simulink model "RB_KAIROS_impControl_compensation"  (R2020b)
settings: Solver=ode4  StartTime=0.0  StopTime=t_end  FixedStep=Ts  RelTol=1e-3
values from neighbouring files (symbols this model uses):
  am = 0.3    [RB_KAIROS_ImpControl_OpSpace_quat_2020b_safety_main.m]
  am_r = 0.3    [RB_KAIROS_ImpControl_OpSpace_quat_2020b_safety_main.m]
  Kc = diag(50*ones(6,1))    [RB_KAIROS_ImpControl_OpSpace_quat_2020b_safety_main.m]
  Kp = 2*[400;400;400;400;0;0;0]    [RB_KAIROS_ImpControl_OpSpace_quat_2020b_safety_main.m]
  Kv = [1000;1000;1000;[300;300;300;300;300;300;300]]    [RB_KAIROS_ImpControl_OpSpace_quat_2020b_safety_main.m]
  model_sample_time = 0.001    [RB_KAIROS_ImpControl_OpSpace_quat_2020b_safety_main.m]
  q_dot_0 = zeros(10,1)    [RB_KAIROS_ImpControl_OpSpace_quat_2020b_safety_main.m]
  T_i = K    [RB_KAIROS_ImpControl_OpSpace_quat_2020b_safety_main.m]
  tau_ext = [0 0 0 0 0 0 0 0 0 0 0]    [RB_KAIROS_ImpControl_OpSpace_quat_2020b_safety_main.m]
  v_SMU = 10    [RB_KAIROS_ImpControl_OpSpace_quat_2020b_safety_main.m]
  vm = 0.5    [RB_KAIROS_ImpControl_OpSpace_quat_2020b_safety_main.m]
  vm_r = 0.5    [RB_KAIROS_ImpControl_OpSpace_quat_2020b_safety_main.m]
undefined symbols (not defined in the file or in its folder): DiscIntNeverNeededParam, magnitude, q_0, T_f
libraries: simulink x4, utils x4, transformations_lib x3
(part 11 of 18)

== matlab function RB_KAIROS_impControl_compensation/CONTROLLER /Kinematics and Dynamics/Dynamics - Configuration space/Arm Gravity terms ==
  data: qv input; G output; qa input; g input
function G = get_G(qv,qa,g)
%GET_G
%    G = GET_G(qv,qa,G)

%    This function was generated by the Symbolic Math Toolbox version 8.6.
%    14-Feb-2023 10:02:51

q2 = qa(2);
q3 = qa(3);
q4 = qa(4);
q5 = qa(5);
q6 = qa(6);
q7 = qa(7);
t2 = cos(q2);
t3 = cos(q3);
t4 = cos(q4);
t5 = cos(q5);
t6 = cos(q6);
t7 = cos(q7);
t8 = sin(q2);
t9 = sin(q3);
t10 = sin(q4);
t11 = sin(q5);
t12 = sin(q6);
t13 = sin(q7);
t14 = t2.*t4;
t15 = t2.*t10;
t16 = t4.*t8;
t17 = t8.*t10;
t18 = t8.*t9.*t11;
t22 = t2.*t5.*t9;
t23 = t3.*t5.*t8;
t25 = t2.*t9.*t11;
t26 = t3.*t8.*t11;
t27 = t5.*t8.*t9;
t35 = t8.*(7.9e+1./2.5e+2);
t36 = t2.*t3.*(3.3e+1./4.0e+2);
t40 = t8.*t9.*(3.3e+1./4.0e+2);
t19 = t3.*t14;
t20 = t3.*t15;
t21 = t3.*t16;
t24 = t3.*t17;
t28 = t5.*t9.*t16;
t29 = t9.*t11.*t16;
t32 = t9.*t12.*t17;
t33 = -t25;
t34 = -t27;
t37 = t14.*(3.3e+1./4.0e+2);
t38 = t15.*(4.8e+1./1.25e+2);
t39 = t16.*(4.8e+1./1.25e+2);
t41 = t17.*(3.3e+1./4.0e+2);
t44 = -t40;
t46 = t9.*t17.*(4.8e+1./1.25e+2);
t53 = t9.*t16.*(3.3e+1./4.0e+2);
t30 = -t20;
t31 = -t21;
t42 = -t29;
t43 = -t32;
t45 = -t41;
t47 = t14+t24;
t48 = t17+t19;
t49 = t19.*(3.3e+1./4.0e+2);
t50 = t20.*(4.8e+1./1.25e+2);
t51 = t21.*(4.8e+1./1.25e+2);
t52 = t24.*(3.3e+1./4.0e+2);
t54 = -t46;
t58 = -t53;
t65 = t26+t28;
t55 = -t49;
t56 = -t50;
t57 = -t51;
t59 = t15+t31;
t60 = t16+t30;
t61 = t5.*t48;
t62 = t6.*t47;
t63 = t11.*t48;
t64 = t12.*t47;
t72 = t23+t42;
t73 = t6.*t65;
t66 = t5.*t62;
t67 = t5.*t59;
t68 = -t62;
t69 = t11.*t59;
t70 = t12.*t59;
t71 = t12.*t60;
t75 = t22+t63;
t77 = t33+t61;
t79 = -t6.*(t25-t61);
t82 = t43+t73;
t74 = -t66;
t76 = t18+t67;
t78 = t34+t69;
t85 = t71+t79;
t80 = t6.*t76;
t81 = t12.*t76;
t83 = t70+t74;
t84 = t64+t80;
t86 = t68+t81;
G = [0.0;0.0;0.0;0.0;g.*(t16.*1.0442e-1-t17.*5.317e-2-t19.*5.317e-2-t20.*1.0442e-1+t35+t36+t2.*t9.*2.7454e-2).*(-3.587895)+g.*(t2.*3.141e-3-t8.*2.872e-2).*6.46926e-1+g.*(t16.*(-3.45563e-1)+t20.*3.45563e-1+t22.*4.1065e-2-t25.*1.1953e-2-t35-t36+t41+t49+t61.*1.1953e-2+t63.*4.1065e-2).*1.225946-g.*(t35+t36+t39-t41+t55+t56+t71.*(1.1e+1./1.25e+2)-t6.*t60.*6.1597e-2-t7.*t75.*4.252e-3+t13.*t75.*1.0517e-2+t7.*t85.*1.0517e-2+t13.*t85.*4.252e-3-t6.*(t25-t61).*(1.1e+1./1.25e+2)-t12.*(t25-t61).*6.1597e-2).*7.35522e-1+g.*(t22.*1.0517e-2-t35-t36-t39+t41+t49+t50+t63.*1.0517e-2-t71.*6.0149e-2+t6.*t60.*1.4117e-2+t6.*(t25-t61).*6.0149e-2+t12.*(t25-t61).*1.4117e-2).*1.666555-g.*(t8.*2.49498e-1+t2.*t3.*2.7518e-2-t2.*t9.*3.9252e-2).*3.228604;g.*(t23.*(-4.1065e-2)+t26.*1.1953e-2+t28.*1.1953e-2+t29.*4.1065e-2+t44+t53+t9.*t17.*3.45563e-1).*(-1.225946)+g.*(t3.*t8.*3.9252e-2+t8.*t9.*2.7518e-2).*3.228604-g.*(t44+t3.*t8.*2.7454e-2+t9.*t16.*5.317e-2+t9.*t17.*1.0442e-1).*3.587895-g.*(t32.*(1.1e+1./1.25e+2)+t44+t46+t53-t73.*(1.1e+1./1.25e+2)-t12.*t65.*6.1597e-2-t7.*t72.*4.252e-3+t13.*t72.*1.0517e-2+t7.*(t32-t73).*1.0517e-2+t13.*(t32-t73).*4.252e-3-t6.*t9.*t17.*6.1597e-2).*7.35522e-1+g.*(t23.*1.0517e-2-t29.*1.0517e-2-t32.*6.0149e-2+t40+t54+t58+t73.*6.0149e-2+t12.*t65.*1.4117e-2+t6.*t9.*t17.*1.4117e-2).*1.666555;g.*(t14.*5.317e-2+t15.*1.0442e-1-t21.*1.0442e-1+t24.*5.317e-2).*(-3.587895)-g.*(t37+t38+t52+t57-t66.*6.0149e-2+t70.*6.0149e-2+t11.*t47.*1.0517e-2-t6.*t59.*1.4117e-2-t5.*t64.*1.4117e-2).*1.666555-g.*(t37+t38+t52+t57-t66.*(1.1e+1./1.25e+2)+t70.*(1.1e+1./1.25e+2)-t6.*t59.*6.1597e-2-t5.*t64.*6.1597e-2-t7.*(t66-t70).*1.0517e-2-t13.*(t66-t70).*4.252e-3+t7.*t11.*t47.*4.252e-3-t11.*t13.*t47.*1.0517e-2).*7.35522e-1-g.*(t15.*3.45563e-1-t21.*3.45563e-1+t37+t52+t5.*t47.*1.1953e-2+t11.*t47.*4.1065e-2).*1.225946;g.*(t7.*t76.*(-4.252e-3)+t13.*t76.*1.0517e-2+t6.*(t27-t69).*(1.1e+1./1.25e+2)+t12.*(t27-t69).*6.1597e-2+t6.*t7.*(t27-t69).*1.0517e-2+t6.*t13.*(t27-t69).*4.252e-3).*7.35522e-1-g.*(t18.*1.0517e-2+t67.*1.0517e-2-t6.*(t27-t69).*6.0149e-2-t12.*(t27-t69).*1.4117e-2).*1.666555-g.*(t18.*4.1065e-2+t27.*1.1953e-2+t67.*4.1065e-2-t69.*1.1953e-2).*1.225946;g.*(t62.*(1.1e+1./1.25e+2)+t64.*6.1597e-2+t80.*6.1597e-2-t81.*(1.1e+1./1.25e+2)+t7.*(t62-t81).*1.0517e-2+t13.*(t62-t81).*4.252e-3).*7.35522e-1+g.*(t62.*6.0149e-2+t64.*1.4117e-2+t80.*1.4117e-2-t81.*6.0149e-2).*1.666555;g.*(t7.*t84.*(-4.252e-3)+t13.*t84.*1.0517e-2+t7.*(t27-t69).*1.0517e-2+t13.*(t27-t69).*4.252e-3).*(-7.35522e-1)];

== matlab function RB_KAIROS_impControl_compensation/CONTROLLER /Kinematics and Dynamics/Dynamics - Configuration space/Chassis Coriolis//Centrifugal Matrix  ==
  data: qv input; Cv output; qdv input
function Cv = get_Cv(qv,qdv)
%GET_CV
%    CV = GET_CV(qv,qdv)

%    This function was generated by the Symbolic Math Toolbox version 8.6.
%    17-Apr-2023 16:26:18

phi = qv(3);
phid = qdv(3);
t2 = cos(phi);
t3 = sin(phi);
Cv = reshape([0.0,0.0,0.0,0.0,0.0,0.0,0.0,0.0,0.0,0.0,0.0,0.0,0.0,0.0,phid.*(t2.*5.016614113875+t3.*1.5530402125),phid.*(t2.*2.224265165851475e+15-t3.*7.184797878510198e+15).*(-6.982261990806649e-16),0.0,0.0,0.0,0.0,0.0,0.0,0.0,0.0,0.0,0.0,0.0,0.0,0.0,0.0,0.0,0.0,0.0,0.0,0.0,0.0,0.0,0.0,0.0,0.0,0.0,0.0,0.0,0.0,0.0,0.0,0.0,0.0,0.0],[7,7]);

== matlab function RB_KAIROS_impControl_compensation/CONTROLLER /Kinematics and Dynamics/Dynamics - Configuration space/Chassis Mass Matrix ==
  data: qv input; Mv output
function Mv = get_Mv(qv)
%GET_MV
%    MV = GET_MV(qv)

%    This function was generated by the Symbolic Math Toolbox version 8.6.
%    17-Apr-2023 16:26:18

phi = qv(3);
t2 = cos(phi);
t3 = sin(phi);
t4 = t2.*5.016614113875;
t5 = t2.*1.5530402125;
t6 = t3.*5.016614113875;
t7 = t3.*1.5530402125;
t8 = -t4;
t9 = -t5;
t10 = -t7;
t11 = t6+t9;
t12 = t8+t10;
Mv = reshape([2.0745e+2,0.0,t11,0.0,0.0,0.0,0.0,0.0,2.0745e+2,t12,0.0,0.0,0.0,0.0,t11,t12,7.022445651482428,0.0,0.0,0.0,0.0,0.0,0.0,0.0,1.2499975e-2,0.0,0.0,0.0,0.0,0.0,0.0,0.0,1.2499975e-2,0.0,0.0,0.0,0.0,0.0,0.0,0.0,1.2499975e-2,0.0,0.0,0.0,0.0,0.0,0.0,0.0,1.2499975e-2],[7,7]);

== matlab function RB_KAIROS_impControl_compensation/CONTROLLER /Kinematics and Dynamics/Dynamics - Configuration space/MATLAB Function ==
  data: M_a input; M output; M_v input
function M = combine_M(M_a, M_v)

%nw = number of wheels, nv = DOF of chassis, na = DOF of the arm. Wheels are neglected in this
%case
nw = 4;
nv = size(M_v,1)-nw;
na = size(M_a,1)-nv;

Ma_up = M_a(1:nv, 1:nv); 
Mva = M_a(1:nv, nv+1:nv+na);
Mav = M_a(nv+1:nv+na, 1:nv);
Ma = M_a(nv+1:nv+na, nv+1:nv+na);

Mv = M_v(1:nv, 1:nv);
% Mvw = M_v(1:nv, 4:nv+nw);
% Mwv = M_v(4:nv+nw, 1:nv);
% Mw = M_v(nv+1:nv+nw, nv+1:nv+nw);

%output
M = zeros(nv+na, nv+na);

M(1:nv,1:nv) = Mv+Ma_up;
M(1:nv,nv+1:nv+na) = Mva;
M(nv+1:nv+na,1:nv) = Mav;
M(nv+1:nv+na,nv+1:nv+na) = Ma;

== matlab function RB_KAIROS_impControl_compensation/RB-KAIROS/Get EE pose/get_T_A_EE ==
  data: qv input; T_A_EE output; qa input
function T_A_EE = get_T_A_EE(qv,qa)
%GET_T_A_EE
%    T_A_EE = GET_T_A_EE(qv,qa)

%    This function was generated by the Symbolic Math Toolbox version 8.6.
%    14-Feb-2023 10:02:51

q1 = qa(1);
q2 = qa(2);
q3 = qa(3);
q4 = qa(4);
q5 = qa(5);
q6 = qa(6);
q7 = qa(7);
t2 = cos(q1);
t3 = cos(q2);
t4 = cos(q3);
t5 = cos(q4);
t6 = cos(q5);
t7 = cos(q6);
t8 = cos(q7);
t9 = sin(q1);
t10 = sin(q2);
t11 = sin(q3);
t12 = sin(q4);
t13 = sin(q5);
t14 = sin(q6);
t15 = sin(q7);
t16 = t2.*t4;
t17 = t3.*t5;
t18 = t2.*t11;
t19 = t4.*t9;
t20 = t3.*t12;
t21 = t9.*t11;
t22 = t9.*t10.*t12;
t23 = t10.*t11.*t13;
t27 = t2.*t5.*t10;
t28 = t4.*t5.*t10;
t30 = t2.*t10.*t12;
t31 = t5.*t9.*t10;
t32 = t4.*t10.*t12;
t33 = t6.*t10.*t11;
t24 = t3.*t16;
t25 = t3.*t18;
t26 = t3.*t19;
t29 = t3.*t21;
t35 = -t28;
t37 = -t30;
t38 = -t31;
t39 = -t33;
t42 = t17+t32;
t34 = -t24;
t36 = -t29;
t40 = t18+t26;
t41 = t19+t25;
t45 = t20+t35;
t50 = t14.*t42;
t43 = t16+t36;
t44 = t21+t34;
t46 = t5.*t40;
t47 = t6.*t41;
t48 = t12.*t40;
t49 = t13.*t41;
t54 = t6.*t45;
t57 = t13.*t45;
t51 = t5.*t44;
t52 = t6.*t43;
t53 = -t47;
t55 = t12.*t44;
t56 = t13.*t43;
t59 = t22+t46;
t60 = t38+t48;
t61 = t23+t54;
t65 = t39+t57;
t69 = -t14.*(t31-t48);
t58 = -t52;
t62 = t27+t55;
t63 = t6.*t59;
t64 = t13.*t59;
t66 = t37+t51;
t68 = t7.*t61;
t70 = -t6.*(t30-t51);
t71 = -t13.*(t30-t51);
t67 = t14.*t62;
t72 = t56+t63;
t73 = t50+t68;
t74 = t49+t70;
t75 = t58+t64;
t77 = t53+t71;
t76 = t7.*t72;
t78 = t7.*t74;
t79 = -t76;
t80 = -t78;
t81 = t69+t79;
t82 = t67+t80;
T_A_EE = reshape([t15.*(t47+t13.*(t30-t51))+t8.*t82,t8.*(t76+t14.*(t31-t48))-t15.*(t52-t64),t8.*t73-t15.*(t33-t57),0.0,t8.*(t47+t13.*(t30-t51))-t15.*t82,-t15.*(t76+t14.*(t31-t48))-t8.*(t52-t64),-t15.*t73-t8.*(t33-t57),0.0,-t7.*t62-t14.*t74,t14.*t72-t7.*(t31-t48),-t7.*t42+t14.*t61,0.0,t21.*(-3.3e+1./4.0e+2)+t24.*(3.3e+1./4.0e+2)+t27.*(4.8e+1./1.25e+2)-t30.*(3.3e+1./4.0e+2)+t51.*(3.3e+1./4.0e+2)+t55.*(4.8e+1./1.25e+2)+t67.*(1.1e+1./1.25e+2)-t78.*(1.1e+1./1.25e+2)+t2.*t10.*(7.9e+1./2.5e+2)-t7.*t62.*(1.07e+2./1.0e+3)-t14.*t74.*(1.07e+2./1.0e+3),t18.*(3.3e+1./4.0e+2)-t22.*(3.3e+1./4.0e+2)+t26.*(3.3e+1./4.0e+2)+t31.*(4.8e+1./1.25e+2)-t46.*(3.3e+1./4.0e+2)-t48.*(4.8e+1./1.25e+2)+t76.*(1.1e+1./1.25e+2)+t9.*t10.*(7.9e+1./2.5e+2)+t14.*t72.*(1.07e+2./1.0e+3)-t7.*(t31-t48).*(1.07e+2./1.0e+3)+t14.*(t31-t48).*(1.1e+1./1.25e+2),t3.*(7.9e+1./2.5e+2)+t17.*(4.8e+1./1.25e+2)-t20.*(3.3e+1./4.0e+2)+t28.*(3.3e+1./4.0e+2)+t32.*(4.8e+1./1.25e+2)+t50.*(1.1e+1./1.25e+2)+t68.*(1.1e+1./1.25e+2)-t4.*t10.*(3.3e+1./4.0e+2)-t7.*t42.*(1.07e+2./1.0e+3)+t14.*t61.*(1.07e+2./1.0e+3)+3.33e+2./1.0e+3,1.0],[4,4]);

== matlab function RB_KAIROS_impControl_compensation/RB-KAIROS/Get EE pose/MATLAB Function ==
  data: T_A_EE input; T_W_EE output; qv input
function T_W_EE = forward_kinematics(T_A_EE,qv)
% Computes the forward kinematics of RB-KAIROS. 
% V = Vehicle
% A = Arm
% W = world
% EE = end effector
% e.g. T_V_A is the transformation matrix between the vehicle and the arm

Ab_x = -0.275;
Ab_y = -0.155;
Ab_z = 0.345;
Ab_a = pi;

T_V_A = [ ...
    cos(Ab_a), -sin(Ab_a), 0, Ab_x;
    sin(Ab_a),  cos(Ab_a), 0, Ab_y;
    0,          0,         1, Ab_z;
    0,          0,         0, 1   ];

T_W_V = [ ...
    cos(qv(3)) -sin(qv(3)), 0, qv(1);
    sin(qv(3)),  cos(qv(3)), 0, qv(2);
    0,          0,         1, 0.345;
    0,          0,         0, 1   ];

T_W_EE = T_W_V*T_V_A*T_A_EE;

end

== matlab function RB_KAIROS_impControl_compensation/Trajectory Generator/move2pose/Subsystem/EE to POI ==
  data: p_POI input; transform output
function transform = EE_to_POI(p_POI)

p_scew = [...
0 -p_POI(3) p_POI(2)
p_POI(3) 0 -p_POI(1)
-p_POI(2) p_POI(1) 0];

transform = [...
    eye(3) -p_scew
    zeros(3) eye(3)];

== matlab function RB_KAIROS_impControl_compensation/Trajectory Generator/move2pose/Subsystem/EE to POI2 ==
  data: human_dist input; human output; crit1 input; crit2 input; v_SMU input; v_SMU_inter output; v_max input
function [human,v_SMU_inter] = LinInterpoly(human_dist,crit1,crit2,v_SMU,v_max)

if human_dist > crit2
    v_SMU_inter = v_max;
    human = 0;
elseif human_dist < crit1
    v_SMU_inter = v_SMU;
    human = 1;
else
    human = 1;
    
    slope = (v_max-v_SMU)/(crit2-crit1);
    shift = v_max - crit2*slope;
    
    v_SMU_inter = human_dist*slope+shift;
end

end

== matlab function RB_KAIROS_impControl_compensation/Trajectory Generator/move2pose/Subsystem/POI to EE ==
  data: p_POI input; transform output
function transform = POI_to_EE(p_POI)

p_scew = [...
0 -p_POI(3) p_POI(2)
p_POI(3) 0 -p_POI(1)
-p_POI(2) p_POI(1) 0];

transform = [...
    eye(3) p_scew
    zeros(3) eye(3)];

== matlab function RB_KAIROS_impControl_compensation/CONTROLLER /Kinematics and Dynamics/Dynamics - Configuration space1/MATLAB Function ==
  data: M_a input; M output; M_v input; Mva output
function [M, Mva] = combine_M(M_a, M_v)
%nw = number of wheels, nv = DOF of chassis, na = DOF of the arm. Wheels are neglected in this
%case
nw = 4;
nv = size(M_v,1)-nw;
na = size(M_a,1)-nv;

Ma_up = M_a(1:nv, 1:nv); 
Mva = M_a(1:nv, nv+1:nv+na);
Mav = M_a(nv+1:nv+na, 1:nv);
Ma = M_a(nv+1:nv+na, nv+1:nv+na);

Mv_nowheels = M_v(1:nv, 1:nv);
% Mv_nowheelsw = M_v(1:nv, 4:nv+nw);
% Mwv = M_v(4:nv+nw, 1:nv);
% Mw = M_v(nv+1:nv+nw, nv+1:nv+nw);

%output
M = zeros(nv+na, nv+na);
 
M(1:nv,1:nv) = Mv_nowheels+Ma_up;
M(1:nv,nv+1:nv+na) = Mva;
M(nv+1:nv+na,1:nv) = Mav;
M(nv+1:nv+na,nv+1:nv+na) = Ma;

== matlab function RB_KAIROS_impControl_compensation/CONTROLLER /Kinematics and Dynamics/Dynamics - Configuration space1/MATLAB Function1 ==
  data: C_a input; C output; C_v input; Cva output
function [C, Cva] = combine_C(C_a, C_v)


%nw = number of wheels, nv = DOF of chassis, na = DOF of the arm. Wheels are neglected in this
%case
nw = 4;
nv = size(C_v,1)-nw;
na = size(C_a,1)-nv;

Ca_up = C_a(1:nv, 1:nv); 
Cva = C_a(1:nv, nv+1:nv+na);
Cav = C_a(nv+1:nv+na, 1:nv);
Ca = C_a(nv+1:nv+na, nv+1:nv+na);

Cv_nowheels = C_v(1:nv, 1:nv);
% Cvw = C_v(1:nv, 4:nv+nw);
% Cwv = C_v(4:nv+nw, 1:nv);
% Cw = C_v(nv+1:nv+nw, nv+1:nv+nw);

%output
C = zeros(nv+na, nv+na);

C(1:nv,1:nv) = Cv_nowheels+Ca_up;
C(1:nv,nv+1:nv+na) = Cva;
C(nv+1:nv+na,1:nv) = Cav;
C(nv+1:nv+na,nv+1:nv+na) = Ca;

C(1:nv,1:nv) = Cv_nowheels+Ca_up;
C(1:nv,nv+1:nv+na) = zeros(nv,na);
C(nv+1:nv+na,1:nv) = zeros(na,nv);
C(nv+1:nv+na,nv+1:nv+na) = Ca;

%TODO: what about Cv_up??? is it needed or not? Where is it computed

== matlab function RB_KAIROS_impControl_compensation/Trajectory Generator/move2pose/Subsystem/Trajectory Scaling Implementation ==
  data: dX_max input; delta_t input; dX_d_old input; dX_d input; dX_d_new output
function dX_d_new  = velocityShaping_SMU(dX_max,delta_t,dX_d_old, dX_d)
%function [psi,fs,dX_d_new] = velocityShaping_SMU(v_SMU, v_POI, dX_max,human,delta_t,dX_d_old, dX_d)
% Calculate normalized dX_max
if norm(dX_max)~=0
    dX_max = dX_max/norm(dX_max);
else
    dX_max = dX_max*0;
end

% % A constant to adjust the sensitivity of trajectory scaling
% alpha = 1; %alpha = 1/0.95;  %alpha = 0.1;
%     
% % Calculate psi based on v_SMU and v_POI
% psi = 1/alpha*((v_SMU/abs(v_POI(1)))); 
% fs = 1;
%     
% % if  (human<0.5 && dX_max >= v_SMU) 
% if  (human<0.5 && abs(v_POI(1)) >= v_SMU) 
%     if psi<0
%         psi = 0;
%      end
%     % Calculate fs
%     fs = 1/2*(1-cos(pi*psi*delta_t));
% end

%% Franka's limits in the Cartesian space are as follows:

% % % % % % % % % % % % % % % % % % % % % % % % % % % % % % % % % % % % % %  
% %   Name     %  Translation  %  Rotation         %   Elbow            % % 
% % % % % % % % % % % % % % % % % % % % % % % % % % % % % % % % % % % % % %  
% %   dp_max   % 1.7000 ms     %  2.5000 rads      %  2.1750 rads       % %
% %   ddp_max  % 13.0000 ms2   %  25.0000 rads2    %  10.0000 rads2     % %
% %   dddp_max % 6500.0000 ms3 %  12500.0000 rads3 %  5000.0000 rads3   % %
% % % % % % % % % % % % % % % % % % % % % % % % % % % % % % % % % % % % % %
persistent dX_d_limit;
dX_d_limit = [13.0*10^3 + delta_t*dX_d_old(1:3);    25.0*10^3 + delta_t*dX_d_old(4:6)];
if (dX_d < dX_d_limit)
    dX_d_new = dX_d;
else
    dX_d_new = dX_d_limit;
end

== matlab function RB_KAIROS_impControl_compensation/CONTROLLER /Kinematics and Dynamics/Kinematics - error representation/Compute J_x_dot/S(omega) ==
  data: v input; S output
function S = calc_skewsymm(v)

S = [0 -v(3) v(2);
    v(3) 0 -v(1);
    -v(2) v(1) 0];

== matlab function RB_KAIROS_impControl_compensation/CONTROLLER /Kinematics and Dynamics/Kinematics - error representation/Compute J_x_dot/Augment matrix ==
  data: M input; M_aug output
function M_aug = augment_matrix(M)

M_aug = [M, zeros(3,3);
             zeros(3,3), M];

== matlab function RB_KAIROS_impControl_compensation/CONTROLLER /Kinematics and Dynamics/Kinematics - error representation/Compute J_x_dot/MATLAB Function ==
  data: qv input; J_dot output; qa input; qv_dot input; qa_dot input
function J_dot = calc_J_derivative(qv,qa,qv_dot,qa_dot)

qa1 = qa(1);
qa2 = qa(2);
qa3 = qa(3);
qa4 = qa(4);
qa5 = qa(5);
qa6 = qa(6);
qv3= qv(3);

% from Ahmed, S. (1992). Issues in the repeatability of redundant manipulator control : pseudoinverse drift and algorithmic singularities
% The following line computes a 3D matrix, each layer k is the derivative of
% the Jacobian w.r.t. the k-eith joint variable

J_grad = J_gradient(qa1,qa2,qa3,qa4,qa5,qa6,qv3);

% Exploiting dJ/dt = grad(J)*dq/dt, we can multiply each layer by the joint
% velocitites to get the derivative of the Jacobian
J_dot = zeros(6,length(qv)+length(qa));
for i = 1:size(J_grad,3)
J_dot(:,i) = J_grad(:,:,i)*[qv_dot;qa_dot];

end
end

== matlab function RB_KAIROS_impControl_compensation/CONTROLLER /Kinematics and Dynamics/Dynamics - Configuration space/MATLAB Function1 ==
  data: C_a input; C output; C_v input
function C = combine_C(C_a, C_v)


%nw = number of wheels, nv = DOF of chassis, na = DOF of the arm. Wheels are neglected in this
%case
nw = 4;
nv = size(C_v,1)-nw;
na = size(C_a,1)-nv;

Ca_up = C_a(1:nv, 1:nv); 
Cva = C_a(1:nv, nv+1:nv+na);
Cav = C_a(nv+1:nv+na, 1:nv);
Ca = C_a(nv+1:nv+na, nv+1:nv+na);

Cv = C_v(1:nv, 1:nv);
% Cvw = C_v(1:nv, 4:nv+nw);
% Cwv = C_v(4:nv+nw, 1:nv);
% Cw = C_v(nv+1:nv+nw, nv+1:nv+nw);

%output
C = zeros(nv+na, nv+na);

C(1:nv,1:nv) = Cv+Ca_up;
C(1:nv,nv+1:nv+na) = Cva;
C(nv+1:nv+na,1:nv) = Cav;
C(nv+1:nv+na,nv+1:nv+na) = Ca;


%TODO: what about Cv_up??? is it needed or not? Where is it computed

== matlab function RB_KAIROS_impControl_compensation/Trajectory Generator/move2pose/Subsystem/fs_function ==
  data: t input; T input; psi input; time_factor output; Gamma input; Theta input; k input; interpoly input
function time_factor = fs_function_time(t, T, psi, Gamma, Theta, k, interpoly)
%FS_FUNCTION_TIME computes the scaling factor for the next timestep. It is 
% similar to equotation (14) of the reference, except that Theta adds a
% parameter for smoother decline and it allows a slower decline. This is
% achieved by the introduction of time t and setting a duration T for the
% adaption. Phi function underneath is similar to (16) of the reference.
%
% Reference:
% [1] S. Haddadin, A. Albu-Schäffer, A. De Luca, and G. Hirzinger, 
% "Collision detection and reaction: A contribution to safe physical 
% human-robot interaction,” International Conference on Intelligent Robots 
% and Systems, pp. 3356–3363, 2008.
%
% Input variables
% t           = Current runtime
% T           = Duration of adaption
% psi         = Scaling factor for time; 0=No scaling; Theta=stop;
%               >Theta+Gamma = revert motion
% Gamma       = Optional dead-zone between stop and reverting motion (set 0
%               for deactivation)
% Theta       = Optional smoothness or strechting(set 1 for deactivation) 
% k           = speed factor for pushing back; 1=deactivated; the higher 
%               the faster the reverting motion
% interpoly   = Which interpolation to use
%
% Output variables
% time_factor = Factor for scaling the next time increment; 0=Stop motion;
%               1= Normal speed; negative values = revert motion
    
%% Initialize persistent variables for adaption motion
persistent psi_1 adpt ti psi_i
if isempty(psi_1)
    psi_1 = psi;    %remembers the psi from last run
end
if isempty(adpt)
    adpt = false;   %stores if an adaption motion is activated
end
if isempty(ti)
    ti = 0;         %Initial time step for adaption motion
end
if isempty(psi_i)
    psi_i = 0;      %Initial psi for adaption motion
end

% needed to delay tanhlog with one timestep
tanhlog_delay = 0;

%% This If runs only for one timestep!!!
% If current psi is unequal to old one 
% Not directly at the beginning
% Dont start new while a adaption is still running, to prevent reset of
%   initial values
if abs(psi-psi_1)>1e-6 && t>0.001 && adpt==false                          
    adpt=true;          % Activate adaption
    ti=t;               % Set initial timestep to current step

    %%% inital set of position, velo, acceleration for adaption motion 
    psi_i = psi_1;
    tanhlog_delay = 1;    
end

%% If adaption motion needed
if adpt == true 

    %%% calculate the adaption psi, which takes time from ti to
    % ti+T. t is the current runtime, _i initial values, _f final
    % values, _m maximum values

    switch interpoly
        case 0
            adpt=false;         %no adatption  
            psi_adpt = psi;
        case 1
            if tanhlog_delay == 1
                psi_adpt = psi_i;
                tanhlog_delay = 0;
            else
                psi_adpt = tanhlog(t-ti,T,psi_i,psi);  %tanhlog
            end
        case 2
            psi_adpt = cosine(t-ti,T,psi_i,psi);   %Cosine version
        case 3
            psi_adpt = poly3(t-ti,T,psi_i,psi);    %poly3
        case 4
            psi_adpt = poly4(t-ti,T,psi_i,psi);    %poly4
        case 5
            psi_adpt = poly5(t-ti,T,psi_i,psi);    %poly5 
        case 6
            psi_adpt = poly6(t-ti,T,psi_i,psi);    %poly6 
        case 7
            psi_adpt = poly7(t-ti,T,psi_i,psi);    %poly7
        case 10
            psi_adpt = tanhmean(t-ti,T,psi_i,psi);    %tanhmean 
        otherwise
            error('Unknown adaption motion');   %rest
    end

    % This computes the time_factor with the standard fs_function, if there is
    % an adaption running
    time_factor = fs_function_lin(psi_adpt, Gamma, Theta, k);

    %if time is equal than the finish time => adaption motion is complete
    %But it is aborted one timestep earlier, since the finish timestep
    %is already computed correctly by the standard interpolator.
    if t>=(ti+T-0.001)  
        adpt=false;     %If adaption finished => reset
    end
    
else %% time_factor without adaption  
    % This computes the time_factor with the standard fs_function, if there is
    % no adaption
    % Linear decline needed here, since smoothness is in time
    time_factor = fs_function_lin(psi, Gamma, Theta, k);
end

psi_1 = psi;  %remember current psi

end

function time_factor = fs_function(psi, Gamma, Theta, k)
%FS_FUNCTION computes the scaling factor for the next timestep. It is 
% similar to equotation (14) of the reference, except that Theta adds a
% parameter for smoother decline. Phi function underneath is similar to
% (16) of the reference.
%
% Reference:
% [1] S. Haddadin, A. Albu-Schäffer, A. De Luca, and G. Hirzinger, 
% "Collision detection and reaction: A contribution to safe physical 
% human-robot interaction,” International Conference on Intelligent Robots 
% and Systems, pp. 3356–3363, 2008.

% Input variables
% psi         = Scaling factor for time; 0=No scaling; Theta=stop;
%               >Theta+Gamma = revert motion
% Gamma       = Optional dead-zone between stop and reverting motion (set 0
%               for deactivation)
% Theta       = Optional smoothness or strechting(set 1 for deactivation) 
% k           = speed factor for pushing back; 1=deactivated; the higher 
%               the faster the reverting motion

% Output variables
% time_factor = Factor for scaling the next time increment; 0=Stop motion;
%               1= Normal speed; negative values = revert motion
       
time_factor = 0;
if 0 <= psi && psi < Theta    %Equ. (14)
    time_factor = phi(psi, Theta);
elseif Theta <= psi && psi <= Theta+Gamma
    time_factor = 0;
elseif Theta+Gamma < psi && psi <= 2*Theta+Gamma
    time_factor = k*phi(psi-Theta-Gamma, Theta)-k;
elseif 2*Theta+Gamma < psi
    time_factor = -k;
else
    error('Trajectory scaling - fs_function: psi wrong (e.g. psi<0)');
end

end

function [psi_smooth] = phi(psi, Theta)
%PHI computes formular (16); smoother decline of factor
%
% Reference:
% [1] S. Haddadin, A. Albu-Schäffer, A. De Luca, and G. Hirzinger, 
% "Collision detection and reaction: A contribution to safe physical 
% human-robot interaction,” International Conference on Intelligent Robots 
% and Systems, pp. 3356–3363, 2008.
%
% Input variables
% psi     = Scaling factor for time (could be vector to here)
% Theta   = Optional smoothness or strechting(set 1 for deactivation)
%
% Output variables
% psi_smooth = smoother psi value

psi_smooth = 0.5.*(ones(size(psi))+cos((1/Theta)*pi.*psi)); %Equ. (16)

end

function time_factor = fs_function_lin(psi, Gamma, Theta, k)
%FS_FUNCTION_LIN computes the scaling factor for the next timestep. It is 
% similar to equotation (14) of the reference, except that Theta adds a
% parameter for smoother decline. Phi function underneath is linear decline
%
% Reference:
% [1] S. Haddadin, A. Albu-Schäffer, A. De Luca, and G. Hirzinger, 
% "Collision detection and reaction: A contribution to safe physical 
% human-robot interaction,” International Conference on Intelligent Robots 
% and Systems, pp. 3356–3363, 2008.

% Input variables
% psi         = Scaling factor for time; 0=No scaling; Theta=stop;
%               >Theta+Gamma = revert motion
% Gamma       = Optional dead-zone between stop and reverting motion (set 0
%               for deactivation)
% Theta       = Optional smoothness or strechting(set 1 for deactivation) 
% k           = speed factor for pushing back; 1=deactivated; the higher 
%               the faster the reverting motion

% Output variables
% time_factor = Factor for scaling the next time increment; 0=Stop motion;
%               1= Normal speed; negative values = revert motion
       
time_factor = 0;
if 0 <= psi && psi < Theta    %Equ. (14)
    time_factor = lin(psi, Theta);
elseif Theta <= psi && psi <= Theta+Gamma
    time_factor = 0;
elseif Theta+Gamma < psi && psi <= 2*Theta+Gamma
    time_factor = k*lin(psi-Theta-Gamma, Theta)-k;
elseif 2*Theta+Gamma < psi
    time_factor = -k;
else
    error('Trajectory scaling - fs_function: psi wrong (e.g. psi<0)');
end

end

function [psi_smooth] = lin(psi, Theta)
%LIN computes linear decline of factor. selfmade
%
% Input variables
% psi     = Scaling factor for time (could be vector to here)
% Theta   = Optional smoothness or strechting(set 1 for deactivation)
%
% Output variables
% psi_smooth = smoother psi value

psi_smooth = 1-(psi/Theta);

end

function [psi] = tanhlog(t,T,psi_i,psi_f)
%TANHLOG computes a 2 tanh-log trajectories between initial (_i) 
%values and final (_f) values of psi. The first goes to a virtual line in 
%the middle and the second back to d_psi_f=0.
%taken from Internet

psi_mean = (psi_f+psi_i)/2;             % calculate mean value of inital and final value
virt_slope = (4*psi_mean-4*psi_i)/T;    % define slope of virtual line 
virt_shift = psi_mean - virt_slope*T/2; % compute the shift of the virtual line

if t<=T/2 %first part for inital to virtual
    a = 0;         
    b = psi_i; 
    c = virt_slope;
    d = virt_shift;
    k = d-b;

    x = (a*t+b-c*t-d+k)/(2*k);
    w = (tanh(((log(1-x))^2-(log(x))^2)/3)+1)/2;
    p = tanh((log(2-x)-log(x))*(1-(1/sqrt(2))*(log(2-x)+log(x))))+2*x-1;
    q = tanh((log(x+1)-log(1-x))*(1-(1/sqrt(2))*(log(1-x)+log(x+1))));
    s = p*(1-w)+q*w;

    psi = k*s+c*t+d-k;
else    %second part from virtual to final
    a = virt_slope;
    b = virt_shift;
    c = 0;     
    d = psi_f; 
    k = (d-b)*(1/3); %k has to be computed a bit different. Math...

    x = (a*t+b-c*t-d+k)/(2*k);
    w = (tanh(((log(1-x))^2-(log(x))^2)/3)+1)/2;
    p = tanh((log(2-x)-log(x))*(1-(1/sqrt(2))*(log(2-x)+log(x))))+2*x-1;
    q = tanh((log(x+1)-log(1-x))*(1-(1/sqrt(2))*(log(1-x)+log(x+1))));
    s = p*(1-w)+q*w;

    psi = k*s+c*t+d-k;
end

end

function [psi] = cosine(t,T,psi_i,psi_f)
%COSINE computes a cosine trajectory between initial (_i) 
%values and final (_f) values of psi. t is the time since ti; T the
%duration
   
psi = 0.5*(psi_i+psi_f) + 0.5*(psi_i-psi_f)*cos((pi/T)*t);

end

function [psi] = poly3(t,T,psi_i,psi_f)
%POLY3 computes a polynomial trajectory of degree 3 between initial (_i) 
%values and final (_f) values of psi. selfmade with poly_calc

d_psi_i = 0; %with poly3 an adaption to the velocity of the change of psi would be possible
d_psi_f = 0;

a = [...
 conj(psi_i)
 conj(d_psi_i)
 (3*conj(psi_f))/T^2 - (2*conj(d_psi_i))/T - conj(d_psi_f)/T - (3*conj(psi_i))/T^2
 conj(d_psi_f)/T^2 + conj(d_psi_i)/T^2 - (2*conj(psi_f))/T^3 + (2*conj(psi_i))/T^3];

psi = a(1)+a(2)*t+a(3)*t^2+a(4)*t^3;

end

function [psi] = poly4(t,T,psi_i,psi_f)
%POLY4 computes a polynomial trajectory of degree 4 between initial (_i) 
%values and final (_f) values of psi. selfmade with poly_calc

d_psi_i = 0; %with poly4 an adaption to the velocity of the change of psi would be possible
d_psi_f = 0;
dd_psi_f = 0;

a = [...
                                                                                                    conj(psi_i)
                                                                                                  conj(d_psi_i)
       conj(dd_psi_f)/2 - (3*conj(d_psi_f))/T - (3*conj(d_psi_i))/T + (6*conj(psi_f))/T^2 - (6*conj(psi_i))/T^2
   (5*conj(d_psi_f))/T^2 + (3*conj(d_psi_i))/T^2 - conj(dd_psi_f)/T - (8*conj(psi_f))/T^3 + (8*conj(psi_i))/T^3
 conj(dd_psi_f)/(2*T^2) - conj(d_psi_i)/T^3 - (2*conj(d_psi_f))/T^3 + (3*conj(psi_f))/T^4 - (3*conj(psi_i))/T^4];

psi = a(1)+a(2)*t+a(3)*t^2+a(4)*t^3+a(5)*t^4;

end

function [psi] = poly5(t,T,psi_i,psi_f)
%POLY4 computes a polynomial trajectory of degree 4 between initial (_i) 
%values and final (_f) values of psi. selfmade with poly_calc

d_psi_i = 0; %with poly4 an adaption to the velocity of the change of psi would be possible
d_psi_f = 0;
dd_psi_i = 0;
dd_psi_f = 0;

a = [...
                                                                                                                                   conj(psi_i)
                                                                                                                                 conj(d_psi_i)
                                                                                                                              conj(dd_psi_i)/2
 conj(dd_psi_f)/(2*T) - (6*conj(d_psi_i))/T^2 - (4*conj(d_psi_f))/T^2 - (3*conj(dd_psi_i))/(2*T) + (10*conj(psi_f))/T^3 - (10*conj(psi_i))/T^3
 (7*conj(d_psi_f))/T^3 + (8*conj(d_psi_i))/T^3 - conj(dd_psi_f)/T^2 + (3*conj(dd_psi_i))/(2*T^2) - (15*conj(psi_f))/T^4 + (15*conj(psi_i))/T^4
   conj(dd_psi_f)/(2*T^3) - (3*conj(d_psi_i))/T^4 - (3*conj(d_psi_f))/T^4 - conj(dd_psi_i)/(2*T^3) + (6*conj(psi_f))/T^5 - (6*conj(psi_i))/T^5];

psi = a(1)+a(2)*t+a(3)*t^2+a(4)*t^3+a(5)*t^4+a(6)*t^5;

end

function [psi] = poly6(t,T,psi_i,psi_f)
%POLY6 computes a polynomial trajectory of degree 6 between initial (_i) 
%values and final (_f) values of psi. j_m is max jerk. selfmade with poly_calc

d_psi_i = 0; %with poly4 an adaption to the velocity of the change of psi would be possible
d_psi_f = 0;
dd_psi_i = 0;
dd_psi_f = 0;
j_m = 50;

a = [...
                                                                                                                                                           conj(psi_i)
                                                                                                                                                         conj(d_psi_i)
                                                                                                                                                      conj(dd_psi_i)/2
                                                                                                                                                           conj(j_m)/6
      conj(dd_psi_f)/(2*T^2) - (10*conj(d_psi_i))/T^3 - (5*conj(d_psi_f))/T^3 - (3*conj(dd_psi_i))/T^2 - conj(j_m)/(2*T) + (15*conj(psi_f))/T^4 - (15*conj(psi_i))/T^4
        (9*conj(d_psi_f))/T^4 + (15*conj(d_psi_i))/T^4 - conj(dd_psi_f)/T^3 + (4*conj(dd_psi_i))/T^3 + conj(j_m)/(2*T^2) - (24*conj(psi_f))/T^5 + (24*conj(psi_i))/T^5
 conj(dd_psi_f)/(2*T^4) - (6*conj(d_psi_i))/T^5 - (4*conj(d_psi_f))/T^5 - (3*conj(dd_psi_i))/(2*T^4) - conj(j_m)/(6*T^3) + (10*conj(psi_f))/T^6 - (10*conj(psi_i))/T^6];

psi = a(1)+a(2)*t+a(3)*t^2+a(4)*t^3+a(5)*t^4+a(6)*t^5+a(7)*t^6;

end

function [psi] = poly7(t,T,psi_i,psi_f)
%POLY6 computes a polynomial trajectory of degree 6 between initial (_i) 
%values and final (_f) values of psi. j_m is max jerk. selfmade with poly_calc

d_psi_i = 0; %with poly4 an adaption to the velocity of the change of psi would be possible
d_psi_f = 0;
dd_psi_i = 0;
dd_psi_f = 0;
ddd_psi_i = 0;
ddd_psi_f = 0;

a = [...
                                                                                                                                                                                                       conj(psi_i)
                                                                                                                                                                                                     conj(d_psi_i)
                                                                                                                                                                                                  conj(dd_psi_i)/2
                                                                                                                                                                                                 conj(ddd_psi_i)/6
           (5*conj(dd_psi_f))/(2*T^2) - (20*conj(d_psi_i))/T^3 - (15*conj(d_psi_f))/T^3 - (5*conj(dd_psi_i))/T^2 - conj(ddd_psi_f)/(6*T) - (2*conj(ddd_psi_i))/(3*T) + (35*conj(psi_f))/T^4 - (35*conj(psi_i))/T^4
                  (39*conj(d_psi_f))/T^4 + (45*conj(d_psi_i))/T^4 - (7*conj(dd_psi_f))/T^3 + (10*conj(dd_psi_i))/T^3 + conj(ddd_psi_f)/(2*T^2) + conj(ddd_psi_i)/T^2 - (84*conj(psi_f))/T^5 + (84*conj(psi_i))/T^5
 (13*conj(dd_psi_f))/(2*T^4) - (36*conj(d_psi_i))/T^5 - (34*conj(d_psi_f))/T^5 - (15*conj(dd_psi_i))/(2*T^4) - conj(ddd_psi_f)/(2*T^3) - (2*conj(ddd_psi_i))/(3*T^3) + (70*conj(psi_f))/T^6 - (70*conj(psi_i))/T^6
               (10*conj(d_psi_f))/T^6 + (10*conj(d_psi_i))/T^6 - (2*conj(dd_psi_f))/T^5 + (2*conj(dd_psi_i))/T^5 + conj(ddd_psi_f)/(6*T^4) + conj(ddd_psi_i)/(6*T^4) - (20*conj(psi_f))/T^7 + (20*conj(psi_i))/T^7];

psi = a(1)+a(2)*t+a(3)*t^2+a(4)*t^3+a(5)*t^4+a(6)*t^5+a(7)*t^6+a(8)*t^7;

end

function [psi] = tanhmean(t,T,psi_i,psi_f)
%TANHMEAN computes a tanh trajectory between initial (_i) 
%values and final (_f) values of psi. theta is the slope of the transition
%selfmade
                     
t_norm = t/T; %Normalized time necessary for this function
theta = 4;

psi = 0.5*(psi_i+psi_f) + 0.5*(psi_f-psi_i)*tanh(theta*(t_norm-0.5));

end

== matlab function RB_KAIROS_impControl_compensation/Trajectory Generator/move2pose/Subsystem/psi_velocity ==
  data: v_desired input; psi output; v_safe input
function psi  = psi_velocity(v_desired, v_safe)
%PSI_VELOCITY Computes a psi value from the comparison of two
%velocities. v_desired is the velocity the robot should move and v_safe
%sets an upper limit. The returned psi value scales down the velocity to a 
%safe value. Both values can be vectors, then the function checks the psi
%value for each dimension and returns the most restrictive psi (=highest).
%
% Input variables
% v_desired = The velocity the robot should move with
% v_safe    = The maximal velocity which is safe for this movement
%
% Output variables
% psi       = value for influencing the speed of the robot

psi = 0;
n = size(v_desired,2);  %n= dimension of velocity
psis = zeros(n,1);      %predefine vector for each dimension
for i=1:n               %Check each dimension
    psis(i) = psi_velocity_single(v_desired(i), v_safe(i));
end

psi = max(psis);        %Take most restrictive psi for all dimensions

end

function [psi_single] = psi_velocity_single(v_desired, v_safe)
%PSI_VELOCITY_SINGLE Computes a psi value from the comparison of two
%velocities. v_desired is the velocity the robot should move and v_safe
%sets an upper limit. The returned psi value scales down the velocity to a 
%safe value, if v_desired is greater than v_safe. This function compares
%only one dimension.
%
% Input variables
% v_desired  = The velocity the robot should move with
% v_safe     = The maximal velocity which is safe for this movement
%
% Output variables
% psi_single = value for influencing the speed of the robot

psi_single = 0;
if v_desired <= v_safe                   %No danger
    psi_single = 0;                     %=> No scaling
elseif v_desired > v_safe              %Desired velocity is dangerous
	psi_single = (1-(v_safe/v_desired));%=> Scaling of time to safe velocity
end

end
